simulink model "ChiefMaster_TTC580"  (R2022b)
settings: Solver=FixedStepAuto  StartTime=0.0  StopTime=10  FixedStep=0.01  RelTol=1e-3
values from neighbouring files (symbols this model uses):
  BattBox1_No = single(1)    [Parameters.m]
  BattBox2_No = single(2)    [Parameters.m]
  BattBox3_No = single(3)    [Parameters.m]
  CurrentLB = single(-3)    [Parameters.m]
  CurrentReductionConstant_Lvl0 = single(0.03)    [Parameters.m]
  CurrentReductionConstant_Lvl1 = single(0.05)    [Parameters.m]
  CurrentReductionConstant_Lvl2 = single(0.07)    [Parameters.m]
  CurrentReductionConstant_Lvl3 = single(0.1)    [Parameters.m]
  CurrentUB = single(3)    [Parameters.m]
  DCHV_Minus_In_Delay_ms = single(500)    [Parameters.m]
  FL_sHVC_CellBalanceVoltage_mV = single(3500)    [Parameters.m]
  FL_sInrushCurrent_dividebyzero = single(0.00001)    [Parameters.m]
  FL_u8HMI_BuzzerTimer = uint8(3)    [Parameters.m]
  IP_boActValue = true    [Parameters.m]
  IP_boDeactValue = false    [Parameters.m]
  IP_boInitValue = false    [Parameters.m]
  IP_s_LB = 18000    [Parameters.m]
  IP_s_UB = 22000    [Parameters.m]
  IP_sBatt1_ChargeCurrentMax_Factor = single(0.1)    [Parameters.m]
  IP_sBatt1_ChargeCurrentMax_LB = single(0)    [Parameters.m]
  IP_sBatt1_ChargeCurrentMax_Offset = single(0)    [Parameters.m]
  IP_sBatt1_ChargeCurrentMax_UB = single(6553.5)    [Parameters.m]
  IP_sBatt1_Current_Factor = single(0.1)    [Parameters.m]
  IP_sBatt1_Current_LB = single(-3276.8)    [Parameters.m]
  IP_sBatt1_Current_Offset = single(0)    [Parameters.m]
  IP_sBatt1_Current_UB = single(3276.8)    [Parameters.m]
  IP_sBatt1_DisChargeCurrentMax_Factor = single(0.1)    [Parameters.m]
  IP_sBatt1_DisChargeCurrentMax_LB = single(0)    [Parameters.m]
  IP_sBatt1_DisChargeCurrentMax_Offset = single(0)    [Parameters.m]
  IP_sBatt1_DisChargeCurrentMax_UB = single(6553.5)    [Parameters.m]
  IP_sBatt1_InsulationResistance_Factor = single(5)    [Parameters.m]
  IP_sBatt1_InsulationResistance_LB = single(0)    [Parameters.m]
  IP_sBatt1_InsulationResistance_Offset = single(0)    [Parameters.m]
  IP_sBatt1_InsulationResistance_UB = single(0)    [Parameters.m]
  IP_sBatt1_LiBa_IntResist_mOhm = single(25)    [Parameters.m]
  IP_sBatt1_SOC_Factor = single(1)    [Parameters.m]
  IP_sBatt1_SOC_LB = single(0)    [Parameters.m]
  IP_sBatt1_SOC_Offset = single(0)    [Parameters.m]
  IP_sBatt1_SOC_UB = single(100)    [Parameters.m]
  IP_sBatt1_SOH_Factor = single(1)    [Parameters.m]
  IP_sBatt1_SOH_LB = single(0)    [Parameters.m]
  IP_sBatt1_SOH_Offset = single(0)    [Parameters.m]
  IP_sBatt1_SOH_UB = single(100)    [Parameters.m]
  IP_sBatt1_Ubatt_Factor = single(0.1)    [Parameters.m]
  IP_sBatt1_Ubatt_LB = single(0)    [Parameters.m]
  IP_sBatt1_Ubatt_Offset = single(0)    [Parameters.m]
  IP_sBatt1_Ubatt_UB = single(6553.5)    [Parameters.m]
  IP_sBatt1_UserRi_Factor = single(1)    [Parameters.m]
  IP_sBatt1_UserRi_LB = single(0)    [Parameters.m]
  IP_sBatt1_UserRi_Offset = single(0)    [Parameters.m]
  IP_sBatt1_UserRi_UB = single(255)    [Parameters.m]
  IP_sBatt1_VoltageAtSensor_Factor = single(0.02)    [Parameters.m]
  IP_sBatt1_VoltageAtSensor_LB = single(0)    [Parameters.m]
  IP_sBatt1_VoltageAtSensor_Offset = single(0)    [Parameters.m]
  IP_sBatt1_VoltageAtSensor_UB = single(1310.7)    [Parameters.m]
  IP_sBatt2_LiBa_IntResist_mOhm = single(25)    [Parameters.m]
  IP_sBatt3_LiBa_IntResist_mOhm = single(25)    [Parameters.m]
  IP_sEM_LB = 2000    [Parameters.m]
  IP_sEM_UB = 8000    [Parameters.m]
  IP_sFB_LB = 5000    [Parameters.m]
  IP_sFB_UB = 10000    [Parameters.m]
  IP_sHVIL_LB = 12000    [Parameters.m]
  IP_sHVIL_UB = 15000    [Parameters.m]
  IP_sLoad_Voltage_Factor = single(1)    [Parameters.m]
  IP_sLoad_Voltage_LB = single(0)    [Parameters.m]
  IP_sLoad_Voltage_Offset = single(0)    [Parameters.m]
  IP_sLoad_Voltage_UB = single(65535)    [Parameters.m]
  IP_u8HVIL_Delay_ms = uint8(100)    [Parameters.m]
  IP_u8HW_IN_delay_ms = uint8(100)    [Parameters.m]
  IT_sInsulationSafeValue_kOhm = single(650)    [Parameters.m]
  IT_u8IMD_DelayTime_s = uint8(20)    [Parameters.m]
  MainHV_Minus_In_Delay = single(5)    [Parameters.m]
  MainHV_StatusDelay = single(5)    [Parameters.m]
  NotAvailable_uint16 = single(65535)    [Parameters.m]
  NotAvailable_uint8 = uint8(255)    [Parameters.m]
  OP_boHVIL_Supply = boolean(1)    [Parameters.m]
  SafeCurrentToCloseHV_A = single(5)    [Parameters.m]
  SafeVoltageToCloseHV_V = single(0.5)    [Parameters.m]
  UnexpectedBattChargingFcn_Available = boolean(1)    [Parameters.m]
  Voltage_NA_UB = uint16(65535)    [Parameters.m]
  VoltageSensorAvailableBB1 = boolean(0)    [Parameters.m]
  VoltageSensorAvailableBB2 = boolean(0)    [Parameters.m]
  VoltageSensorAvailableBB3 = boolean(0)    [Parameters.m]
libraries: simulink x184, Library_DataProcessing_v1_1 x167, Library_DataProcessing_v1 x142, libCM x28
(part 12 of 19)

== system ChiefMaster_TTC580/ChiefMaster/Input Translation/Battery Signals/Subsystem10/Subsystem3 ==
  <IP_boBatt1_IMD_Active : Inport
  "IMD_Req_Databus  " : Inport  Port=2
  Bus Selector : BusSelector  OutputSignals=FL_IMD_Control_Databus.FL_boREQ_IMD_ON_BB1
  Constant : Constant  Value=0  OutDataTypeStr=boolean
  Delay : Delay  DelayLength=3
  Multiport Switch : MultiPortSwitch  DataPortForDefault=Additional data port  DiagnosticForDefault=Warning  SaturateOnIntegerOverflow=off  InputSameDT=off
  IP_boBMS_IMD_Active_BB1 : Outport  OutDataTypeStr=boolean
  wires:
  Multiport Switch/1 -> IP_boBMS_IMD_Active_BB1/1  "IP_boBMS_IMD_Active_BB1"
  <IP_boBatt1_IMD_Active/1 -> Multiport Switch/2
  [Select_Battery1] -> Multiport Switch/1
  Delay/1 -> Multiport Switch/3
  Constant/1 -> Multiport Switch/4, Multiport Switch/5
  "IMD_Req_Databus  "/1 -> Bus Selector/1
  Bus Selector/1 -> Delay/1  "<FL_boREQ_IMD_ON_BB1>"

== system ChiefMaster_TTC580/ChiefMaster/Input Translation/Battery Signals/Subsystem11/Subsystem1 ==
  <IP_sBatt2_UserRi_mOhms_DataBus> : Inport
  Bus Selector7 : BusSelector  OutputSignals=sData
  Constant : Constant  Value=0  OutDataTypeStr=single
  Constant1 : Constant  Value=IP_sBatt2_LiBa_IntResist_mOhm  OutDataTypeStr=single
  Multiport Switch : MultiPortSwitch  DataPortForDefault=Additional data port  DiagnosticForDefault=Warning  SaturateOnIntegerOverflow=off  InputSameDT=off
  IP_sBMS_InternalResistance_BB2 : Outport
  wires:
  Constant1/1 -> Multiport Switch/3
  <IP_sBatt2_UserRi_mOhms_DataBus>/1 -> Bus Selector7/1
  Multiport Switch/1 -> IP_sBMS_InternalResistance_BB2/1  "IP_sBMS_InternalResistance_BB2"
  [Select_Battery2] -> Multiport Switch/1
  Constant/1 -> Multiport Switch/5, Multiport Switch/4
  Bus Selector7/1 -> Multiport Switch/2  "<sData>"

== system ChiefMaster_TTC580/ChiefMaster/Input Translation/Battery Signals/Subsystem11/Subsystem2 ==
  <IP_sBatt3_UserRi_mOhms_DataBus> : Inport
  Bus Selector7 : BusSelector  OutputSignals=sData
  Constant : Constant  Value=0  OutDataTypeStr=single
  Constant1 : Constant  Value=IP_sBatt3_LiBa_IntResist_mOhm  OutDataTypeStr=single
  Multiport Switch : MultiPortSwitch  DataPortForDefault=Additional data port  DiagnosticForDefault=Warning  SaturateOnIntegerOverflow=off  InputSameDT=off
  IP_sBMS_InternalResistance_BB3 : Outport
  wires:
  Bus Selector7/1 -> Multiport Switch/2  "<sData>"
  Constant/1 -> Multiport Switch/4, Multiport Switch/5
  [Select_Battery3] -> Multiport Switch/1
  Multiport Switch/1 -> IP_sBMS_InternalResistance_BB3/1  "IP_sBMS_InternalResistance_BB3"
  <IP_sBatt3_UserRi_mOhms_DataBus>/1 -> Bus Selector7/1
  Constant1/1 -> Multiport Switch/3

== system ChiefMaster_TTC580/ChiefMaster/Input Translation/Battery Signals/Subsystem11/Subsystem3 ==
  <IP_sBatt1_UserRi_mOhms_DataBus> : Inport
  Bus Selector7 : BusSelector  OutputSignals=sData
  Constant : Constant  Value=0  OutDataTypeStr=single
  Constant1 : Constant  Value=IP_sBatt1_LiBa_IntResist_mOhm  OutDataTypeStr=single
  Multiport Switch : MultiPortSwitch  DataPortForDefault=Additional data port  DiagnosticForDefault=Warning  SaturateOnIntegerOverflow=off  InputSameDT=off
  IP_sBMS_InternalResistance_BB1 : Outport
  wires:
  Bus Selector7/1 -> Multiport Switch/2  "<sData>"
  Constant/1 -> Multiport Switch/4, Multiport Switch/5
  [Select_Battery1] -> Multiport Switch/1
  Multiport Switch/1 -> IP_sBMS_InternalResistance_BB1/1  "IP_sBMS_InternalResistance_BB1"
  <IP_sBatt1_UserRi_mOhms_DataBus>/1 -> Bus Selector7/1
  Constant1/1 -> Multiport Switch/3

== system ChiefMaster_TTC580/ChiefMaster/Input Translation/Battery Signals/Subsystem12/Subsystem1 ==
  <IP_sBatt2_InsulationResistance_kOhms_DataBus> : Inport
  <IP_LB_BMS_Pack_Leak_Pos_Raw_mV_DataBus> : Inport  Port=2
  <IP_LB_BMS_Pack_Leak_Neg_Raw_mV_DataBus> : Inport  Port=3
  <IP_LB_BMS_Pack_V_Cells_DataBus> : Inport  Port=4
  Bus Selector : BusSelector  OutputSignals=sData
  Constant : Constant  Value=0  OutDataTypeStr=single
  Multiport Switch : MultiPortSwitch  DataPortForDefault=Additional data port  DiagnosticForDefault=Warning  SaturateOnIntegerOverflow=off  InputSameDT=off
  Subsystem1 : Subsystem
  IP_boBMS_InsulationResistance_kOhm_BB1 : Outport  OutDataTypeStr=single
  IP_boBMS_InsulationResistance_Minus_kOhm_BB1 : Outport  Port=2  OutDataTypeStr=single
  IP_LiBa_Insulation_OK_BB1 : Outport  Port=3
  wires:
  Bus Selector/1 -> Multiport Switch/2  "<sData>"
  <IP_sBatt2_InsulationResistance_kOhms_DataBus>/1 -> Bus Selector/1
  Multiport Switch/1 -> IP_boBMS_InsulationResistance_kOhm_BB1/1  "IP_boBMS_InsulationResistance_kOhm_B2"
  [Select_Battery2] -> Multiport Switch/1
  <IP_LB_BMS_Pack_V_Cells_DataBus>/1 -> Subsystem1/3(<IP_LB_BMS_Pack_V_Cells_DataBus>)
  Subsystem1/1(IP_sLiBa_InsulationRes_Plus_kOhm) -> Multiport Switch/3
  Constant/1 -> Multiport Switch/4, Multiport Switch/5
  <IP_LB_BMS_Pack_Leak_Pos_Raw_mV_DataBus>/1 -> Subsystem1/1(<IP_LB_BMS_Pack_Leak_Pos_Raw_mV_DataBus>)
  <IP_LB_BMS_Pack_Leak_Neg_Raw_mV_DataBus>/1 -> Subsystem1/2(<IP_LB_BMS_Pack_Leak_Neg_Raw_mV_DataBus>)
  Subsystem1/2(IP_sLiBa_InsulationRes_Minus_kOhm) -> IP_boBMS_InsulationResistance_Minus_kOhm_BB1/1
  Subsystem1/3(IP_LiBa_Insulation_Ok_Batt) -> IP_LiBa_Insulation_OK_BB1/1

== system ChiefMaster_TTC580/ChiefMaster/Input Translation/Battery Signals/Subsystem12/Subsystem2 ==
  <IP_sBatt3_InsulationResistance_kOhms_DataBus> : Inport
  <IP_LB_BMS_Pack_Leak_Pos_Raw_mV_DataBus> : Inport  Port=2
  <IP_LB_BMS_Pack_Leak_Neg_Raw_mV_DataBus> : Inport  Port=3
  <IP_LB_BMS_Pack_V_Cells_DataBus> : Inport  Port=4
  Bus Selector : BusSelector  OutputSignals=sData
  Constant : Constant  Value=0  OutDataTypeStr=single
  Multiport Switch : MultiPortSwitch  DataPortForDefault=Additional data port  DiagnosticForDefault=Warning  SaturateOnIntegerOverflow=off  InputSameDT=off
  Subsystem1 : Subsystem
  IP_boBMS_InsulationResistance_kOhm_B3 : Outport  OutDataTypeStr=single
  IP_sLiBa_InsulationRes_Minus_BB3_kOhm : Outport  Port=2  OutDataTypeStr=single
  IP_LiBa_Insulation_Ok_Batt3 : Outport  Port=3
  wires:
  <IP_LB_BMS_Pack_Leak_Pos_Raw_mV_DataBus>/1 -> Subsystem1/1(<IP_LB_BMS_Pack_Leak_Pos_Raw_mV_DataBus>)
  Constant/1 -> Multiport Switch/5, Multiport Switch/4
  Subsystem1/1(IP_sLiBa_InsulationRes_Plus_kOhm) -> Multiport Switch/3
  <IP_LB_BMS_Pack_V_Cells_DataBus>/1 -> Subsystem1/3(<IP_LB_BMS_Pack_V_Cells_DataBus>)
  [Select_Battery3] -> Multiport Switch/1
  Multiport Switch/1 -> IP_boBMS_InsulationResistance_kOhm_B3/1  "IP_boBMS_InsulationResistance_kOhm_B3"
  <IP_sBatt3_InsulationResistance_kOhms_DataBus>/1 -> Bus Selector/1
  Bus Selector/1 -> Multiport Switch/2  "<sData>"
  <IP_LB_BMS_Pack_Leak_Neg_Raw_mV_DataBus>/1 -> Subsystem1/2(<IP_LB_BMS_Pack_Leak_Neg_Raw_mV_DataBus>)
  Subsystem1/3(IP_LiBa_Insulation_Ok_Batt) -> IP_LiBa_Insulation_Ok_Batt3/1
  Subsystem1/2(IP_sLiBa_InsulationRes_Minus_kOhm) -> IP_sLiBa_InsulationRes_Minus_BB3_kOhm/1

== system ChiefMaster_TTC580/ChiefMaster/Input Translation/Battery Signals/Subsystem12/Subsystem3 ==
  <IP_sBatt1_InsulationResistance_kOhms_DataBus> : Inport
  <IP_LB_BMS_Pack_Leak_Pos_Raw_mV_DataBus> : Inport  Port=2
  <IP_LB_BMS_Pack_Leak_Neg_Raw_mV_DataBus> : Inport  Port=3
  <IP_LB_BMS_Pack_V_Cells_DataBus> : Inport  Port=4
  Bus Selector : BusSelector  OutputSignals=sData
  Constant : Constant  Value=0  OutDataTypeStr=single
  Multiport Switch : MultiPortSwitch  DataPortForDefault=Additional data port  DiagnosticForDefault=Warning  SaturateOnIntegerOverflow=off  InputSameDT=off
  Subsystem1 : Subsystem
  IP_boBMS_InsulationResistance_kOhm_BB1 : Outport  OutDataTypeStr=single
  IP_boBMS_InsulationResistance_Minus_kOhm_BB1 : Outport  Port=2  OutDataTypeStr=single
  IP_LiBa_Insulation_OK_BB1 : Outport  Port=3
  wires:
  <IP_LB_BMS_Pack_Leak_Pos_Raw_mV_DataBus>/1 -> Subsystem1/1(<IP_LB_BMS_Pack_Leak_Pos_Raw_mV_DataBus>)
  Constant/1 -> Multiport Switch/5, Multiport Switch/4
  <IP_LB_BMS_Pack_V_Cells_DataBus>/1 -> Subsystem1/3(<IP_LB_BMS_Pack_V_Cells_DataBus>)
  [Select_Battery1] -> Multiport Switch/1
  Multiport Switch/1 -> IP_boBMS_InsulationResistance_kOhm_BB1/1  "IP_boBMS_InsulationResistance_kOhm_BB1"
  <IP_sBatt1_InsulationResistance_kOhms_DataBus>/1 -> Bus Selector/1
  Bus Selector/1 -> Multiport Switch/2  "<sData>"
  <IP_LB_BMS_Pack_Leak_Neg_Raw_mV_DataBus>/1 -> Subsystem1/2(<IP_LB_BMS_Pack_Leak_Neg_Raw_mV_DataBus>)
  Subsystem1/1(IP_sLiBa_InsulationRes_Plus_kOhm) -> Multiport Switch/3
  Subsystem1/2(IP_sLiBa_InsulationRes_Minus_kOhm) -> IP_boBMS_InsulationResistance_Minus_kOhm_BB1/1  "IP_sLiBa_InsulationRes_Minus_BB1_kOhm"
  Subsystem1/3(IP_LiBa_Insulation_Ok_Batt) -> IP_LiBa_Insulation_OK_BB1/1

== system ChiefMaster_TTC580/ChiefMaster/Input Translation/Battery Signals/Subsystem14/Subsystem1 ==
  <IP_sActia_Batt2_MinCellVolt_DataBus> : Inport
  <IP_LB_BMS_ACT_Cel_mV_Min_DataBus> : Inport  Port=2
  Bus Selector1 : BusSelector  OutputSignals=sData
  Bus Selector7 : BusSelector  OutputSignals=sData
  Constant : Constant  Value=0  OutDataTypeStr=single
  Multiport Switch : MultiPortSwitch  DataPortForDefault=Additional data port  DiagnosticForDefault=Warning  SaturateOnIntegerOverflow=off  InputSameDT=off
  IP_sBMS_MinCellVoltage_BB2 : Outport
  wires:
  Multiport Switch/1 -> IP_sBMS_MinCellVoltage_BB2/1  "IP_sBMS_MinCellVoltage_BB2"
  [Select_Battery2] -> Multiport Switch/1
  Constant/1 -> Multiport Switch/5, Multiport Switch/4
  <IP_sActia_Batt2_MinCellVolt_DataBus>/1 -> Bus Selector1/1
  <IP_LB_BMS_ACT_Cel_mV_Min_DataBus>/1 -> Bus Selector7/1
  Bus Selector7/1 -> Multiport Switch/3  "<sData>"
  Bus Selector1/1 -> Multiport Switch/2  "<sData>"

== system ChiefMaster_TTC580/ChiefMaster/Input Translation/Battery Signals/Subsystem14/Subsystem2 ==
  <IP_sActia_Batt3_MinCellVolt_DataBus> : Inport
  <IP_LB_BMS_ACT_Cel_mV_Min_DataBus> : Inport  Port=2
  Bus Selector1 : BusSelector  OutputSignals=sData
  Bus Selector7 : BusSelector  OutputSignals=sData
  Constant : Constant  Value=0  OutDataTypeStr=single
  Multiport Switch : MultiPortSwitch  DataPortForDefault=Additional data port  DiagnosticForDefault=Warning  SaturateOnIntegerOverflow=off  InputSameDT=off
  IP_sBMS_MinCellVoltage_BB3 : Outport
  wires:
  Bus Selector1/1 -> Multiport Switch/2  "<sData>"
  Bus Selector7/1 -> Multiport Switch/3  "<sData>"
  <IP_LB_BMS_ACT_Cel_mV_Min_DataBus>/1 -> Bus Selector7/1
  <IP_sActia_Batt3_MinCellVolt_DataBus>/1 -> Bus Selector1/1
  Constant/1 -> Multiport Switch/4, Multiport Switch/5
  [Select_Battery3] -> Multiport Switch/1
  Multiport Switch/1 -> IP_sBMS_MinCellVoltage_BB3/1  "IP_sBMS_MinCellVoltage_BB3"

== system ChiefMaster_TTC580/ChiefMaster/Input Translation/Battery Signals/Subsystem14/Subsystem3 ==
  <IP_sActia_Batt1_MinCellVolt_mV_DataBus> : Inport
  <IP_LB_BMS_ACT_Cel_mV_Min_DataBus> : Inport  Port=2
  Bus Selector1 : BusSelector  OutputSignals=sData
  Bus Selector7 : BusSelector  OutputSignals=sData
  Constant : Constant  Value=0  OutDataTypeStr=single
  Multiport Switch : MultiPortSwitch  DataPortForDefault=Additional data port  DiagnosticForDefault=Warning  SaturateOnIntegerOverflow=off  InputSameDT=off
  IP_sBMS_MinCellVoltage_BB1 : Outport
  wires:
  Bus Selector1/1 -> Multiport Switch/2  "<sData>"
  Bus Selector7/1 -> Multiport Switch/3  "<sData>"
  <IP_LB_BMS_ACT_Cel_mV_Min_DataBus>/1 -> Bus Selector7/1
  <IP_sActia_Batt1_MinCellVolt_mV_DataBus>/1 -> Bus Selector1/1
  Constant/1 -> Multiport Switch/4, Multiport Switch/5
  [Select_Battery1] -> Multiport Switch/1
  Multiport Switch/1 -> IP_sBMS_MinCellVoltage_BB1/1  "IP_sBMS_MinCellVoltage_BB1"

== system ChiefMaster_TTC580/ChiefMaster/Input Translation/Battery Signals/Subsystem14/Subsystem4 ==
  <IP_sActia_Batt2_MaxCellVolt_DataBus> : Inport
  <IP_LB_BMS_ACT_Cel_mV_Min_DataBus> : Inport  Port=2
  Bus Selector1 : BusSelector  OutputSignals=sData
  Bus Selector7 : BusSelector  OutputSignals=sData
  Constant : Constant  Value=0  OutDataTypeStr=single
  Multiport Switch : MultiPortSwitch  DataPortForDefault=Additional data port  DiagnosticForDefault=Warning  SaturateOnIntegerOverflow=off  InputSameDT=off
  IP_sBMS_MaxCellVoltage_BB2 : Outport
  wires:
  Bus Selector1/1 -> Multiport Switch/2  "<sData>"
  Bus Selector7/1 -> Multiport Switch/3  "<sData>"
  <IP_LB_BMS_ACT_Cel_mV_Min_DataBus>/1 -> Bus Selector7/1
  <IP_sActia_Batt2_MaxCellVolt_DataBus>/1 -> Bus Selector1/1
  Constant/1 -> Multiport Switch/4, Multiport Switch/5
  [Select_Battery2] -> Multiport Switch/1
  Multiport Switch/1 -> IP_sBMS_MaxCellVoltage_BB2/1  "IP_sBMS_MaxCellVoltage_BB2"

== system ChiefMaster_TTC580/ChiefMaster/Input Translation/Battery Signals/Subsystem14/Subsystem5 ==
  <IP_sActia_Batt3_MaxCellVolt_DataBus> : Inport
  <IP_LB_BMS_ACT_Cel_mV_Min_DataBus> : Inport  Port=2
  Bus Selector1 : BusSelector  OutputSignals=sData
  Bus Selector7 : BusSelector  OutputSignals=sData
  Constant : Constant  Value=0  OutDataTypeStr=single
  Multiport Switch : MultiPortSwitch  DataPortForDefault=Additional data port  DiagnosticForDefault=Warning  SaturateOnIntegerOverflow=off  InputSameDT=off
  IP_sBMS_MaxCellVoltage_BB3 : Outport
  wires:
  Multiport Switch/1 -> IP_sBMS_MaxCellVoltage_BB3/1  "IP_sBMS_MaxCellVoltage_BB3"
  [Select_Battery3] -> Multiport Switch/1
  Constant/1 -> Multiport Switch/5, Multiport Switch/4
  <IP_sActia_Batt3_MaxCellVolt_DataBus>/1 -> Bus Selector1/1
  <IP_LB_BMS_ACT_Cel_mV_Min_DataBus>/1 -> Bus Selector7/1
  Bus Selector1/1 -> Multiport Switch/2  "<sData>"
  Bus Selector7/1 -> Multiport Switch/3  "<sData>"

== system ChiefMaster_TTC580/ChiefMaster/Input Translation/Battery Signals/Subsystem14/Subsystem6 ==
  <IP_sActia_Batt1_MaxCellVolt_DataBus> : Inport
  <IP_LB_BMS_ACT_Cel_mV_Min_DataBus> : Inport  Port=2
  Bus Selector1 : BusSelector  OutputSignals=sData
  Bus Selector7 : BusSelector  OutputSignals=sData
  Constant : Constant  Value=0  OutDataTypeStr=single
  Multiport Switch : MultiPortSwitch  DataPortForDefault=Additional data port  DiagnosticForDefault=Warning  SaturateOnIntegerOverflow=off  InputSameDT=off
  IP_sBMS_MaxCellVoltage_BB1 : Outport
  wires:
  Multiport Switch/1 -> IP_sBMS_MaxCellVoltage_BB1/1  "IP_sBMS_MaxCellVoltage_BB1"
  [Select_Battery1] -> Multiport Switch/1
  Constant/1 -> Multiport Switch/5, Multiport Switch/4
  <IP_sActia_Batt1_MaxCellVolt_DataBus>/1 -> Bus Selector1/1
  <IP_LB_BMS_ACT_Cel_mV_Min_DataBus>/1 -> Bus Selector7/1
  Bus Selector1/1 -> Multiport Switch/2  "<sData>"
  Bus Selector7/1 -> Multiport Switch/3  "<sData>"

== system ChiefMaster_TTC580/ChiefMaster/Input Translation/Battery Signals/Subsystem15/Subsystem1 ==
  <IP_sActia_Batt1_MaxTemp_degC_DataBus> : Inport
  <IP_LB_BMS_ACT_Cel_T_Max_Value_DataBus> : Inport  Port=2
  Bus Selector1 : BusSelector  OutputSignals=sData
  Bus Selector7 : BusSelector  OutputSignals=sData
  Constant : Constant  Value=0  OutDataTypeStr=single
  Multiport Switch : MultiPortSwitch  DataPortForDefault=Additional data port  DiagnosticForDefault=Warning  SaturateOnIntegerOverflow=off  InputSameDT=off
  IP_sBMS_MaxTemp_degC_BB1 : Outport
  wires:
  <IP_LB_BMS_ACT_Cel_T_Max_Value_DataBus>/1 -> Bus Selector1/1
  <IP_sActia_Batt1_MaxTemp_degC_DataBus>/1 -> Bus Selector7/1
  Bus Selector1/1 -> Multiport Switch/3  "<sData>"
  Bus Selector7/1 -> Multiport Switch/2  "<sData>"
  Constant/1 -> Multiport Switch/4, Multiport Switch/5
  [Select_Battery1] -> Multiport Switch/1
  Multiport Switch/1 -> IP_sBMS_MaxTemp_degC_BB1/1  "IP_sBMS_MaxTemp_degC_BB1"

== system ChiefMaster_TTC580/ChiefMaster/Input Translation/Battery Signals/Subsystem15/Subsystem2 ==
  <IP_sActia_Batt2_MinTemp_degC_DataBus> : Inport
  <IP_LB_BMS_ACT_Cel_T_Min_Value_DataBus> : Inport  Port=2
  Bus Selector1 : BusSelector  OutputSignals=sData
  Bus Selector7 : BusSelector  OutputSignals=sData
  Constant : Constant  Value=0  OutDataTypeStr=single
  Multiport Switch : MultiPortSwitch  DataPortForDefault=Additional data port  DiagnosticForDefault=Warning  SaturateOnIntegerOverflow=off  InputSameDT=off
  IP_sBMS_MinTemp_degC_BB2 : Outport
  wires:
  <IP_LB_BMS_ACT_Cel_T_Min_Value_DataBus>/1 -> Bus Selector1/1
  <IP_sActia_Batt2_MinTemp_degC_DataBus>/1 -> Bus Selector7/1
  Bus Selector7/1 -> Multiport Switch/2  "<sData>"
  Bus Selector1/1 -> Multiport Switch/3  "<sData>"
  [Select_Battery2] -> Multiport Switch/1
  Multiport Switch/1 -> IP_sBMS_MinTemp_degC_BB2/1  "IP_sBMS_MinTemp_degC_BB2"
  Constant/1 -> Multiport Switch/4, Multiport Switch/5

== system ChiefMaster_TTC580/ChiefMaster/Input Translation/Battery Signals/Subsystem15/Subsystem3 ==
  <IP_sActia_Batt1_MinTemp_degC_DataBus> : Inport
  <IP_LB_BMS_ACT_Cel_T_Min_Value_DataBus> : Inport  Port=2
  Bus Selector1 : BusSelector  OutputSignals=sData
  Bus Selector7 : BusSelector  OutputSignals=sData
  Constant : Constant  Value=0  OutDataTypeStr=single
  Multiport Switch : MultiPortSwitch  DataPortForDefault=Additional data port  DiagnosticForDefault=Warning  SaturateOnIntegerOverflow=off  InputSameDT=off
  IP_sBMS_MinTemp_degC_BB1 : Outport
  wires:
  Multiport Switch/1 -> IP_sBMS_MinTemp_degC_BB1/1  "IP_sBMS_MinTemp_degC_BB1"
  [Select_Battery1] -> Multiport Switch/1
  Constant/1 -> Multiport Switch/5, Multiport Switch/4
  Bus Selector7/1 -> Multiport Switch/2  "<sData>"
  Bus Selector1/1 -> Multiport Switch/3  "<sData>"
  <IP_sActia_Batt1_MinTemp_degC_DataBus>/1 -> Bus Selector7/1
  <IP_LB_BMS_ACT_Cel_T_Min_Value_DataBus>/1 -> Bus Selector1/1

== system ChiefMaster_TTC580/ChiefMaster/Input Translation/Battery Signals/Subsystem15/Subsystem4 ==
  <IP_sActia_Batt2_MaxTemp_degC_DataBus> : Inport
  <IP_LB_BMS_ACT_Cel_T_Max_Value_DataBus> : Inport  Port=2
  Bus Selector1 : BusSelector  OutputSignals=sData
  Bus Selector7 : BusSelector  OutputSignals=sData
  Constant : Constant  Value=0  OutDataTypeStr=single
  Multiport Switch : MultiPortSwitch  DataPortForDefault=Additional data port  DiagnosticForDefault=Warning  SaturateOnIntegerOverflow=off  InputSameDT=off
  IP_sBMS_MaxTemp_degC_BB2 : Outport
  wires:
  Multiport Switch/1 -> IP_sBMS_MaxTemp_degC_BB2/1  "IP_sBMS_MaxTemp_degC_BB2"
  [Select_Battery2] -> Multiport Switch/1
  Constant/1 -> Multiport Switch/5, Multiport Switch/4
  Bus Selector7/1 -> Multiport Switch/2  "<sData>"
  Bus Selector1/1 -> Multiport Switch/3  "<sData>"
  <IP_sActia_Batt2_MaxTemp_degC_DataBus>/1 -> Bus Selector7/1
  <IP_LB_BMS_ACT_Cel_T_Max_Value_DataBus>/1 -> Bus Selector1/1

== system ChiefMaster_TTC580/ChiefMaster/Input Translation/Battery Signals/Subsystem15/Subsystem5 ==
  <IP_sActia_Batt3_MinTemp_degC_DataBus> : Inport
  <IP_LB_BMS_ACT_Cel_T_Min_Value_DataBus> : Inport  Port=2
  Bus Selector1 : BusSelector  OutputSignals=sData
  Bus Selector7 : BusSelector  OutputSignals=sData
  Constant : Constant  Value=0  OutDataTypeStr=single
  Multiport Switch : MultiPortSwitch  DataPortForDefault=Additional data port  DiagnosticForDefault=Warning  SaturateOnIntegerOverflow=off  InputSameDT=off
  IP_sBMS_MinTemp_degC_BB3 : Outport
  wires:
  Multiport Switch/1 -> IP_sBMS_MinTemp_degC_BB3/1  "IP_sBMS_MinTemp_degC_BB3"
  [Select_Battery3] -> Multiport Switch/1
  Constant/1 -> Multiport Switch/5, Multiport Switch/4
  Bus Selector7/1 -> Multiport Switch/2  "<sData>"
  Bus Selector1/1 -> Multiport Switch/3  "<sData>"
  <IP_sActia_Batt3_MinTemp_degC_DataBus>/1 -> Bus Selector7/1
  <IP_LB_BMS_ACT_Cel_T_Min_Value_DataBus>/1 -> Bus Selector1/1

== system ChiefMaster_TTC580/ChiefMaster/Input Translation/Battery Signals/Subsystem15/Subsystem6 ==
  <IP_sActia_Batt3_MaxTemp_degC_DataBus> : Inport
  <IP_LB_BMS_ACT_Cel_T_Max_Value_DataBus> : Inport  Port=2
  Bus Selector1 : BusSelector  OutputSignals=sData
  Bus Selector7 : BusSelector  OutputSignals=sData
  Constant : Constant  Value=0  OutDataTypeStr=single
  Multiport Switch : MultiPortSwitch  DataPortForDefault=Additional data port  DiagnosticForDefault=Warning  SaturateOnIntegerOverflow=off  InputSameDT=off
  IP_sBMS_MaxTemp_degC_BB3 : Outport
  wires:
  <IP_LB_BMS_ACT_Cel_T_Max_Value_DataBus>/1 -> Bus Selector1/1
  <IP_sActia_Batt3_MaxTemp_degC_DataBus>/1 -> Bus Selector7/1
  Bus Selector1/1 -> Multiport Switch/3  "<sData>"
  Bus Selector7/1 -> Multiport Switch/2  "<sData>"
  Constant/1 -> Multiport Switch/4, Multiport Switch/5
  [Select_Battery3] -> Multiport Switch/1
  Multiport Switch/1 -> IP_sBMS_MaxTemp_degC_BB3/1  "IP_sBMS_MaxTemp_degC_BB3"

== system ChiefMaster_TTC580/ChiefMaster/Input Translation/Battery Signals/Subsystem2/Subsystem ==
  IP_boBatt1_HV_REL_ON : Inport
  IP_LB_BMS_IO_state_Input_DataBus : Inport  Port=2
  Bus Selector : BusSelector  OutputSignals=sData
  Compare To Constant : simulink/Logic and Bit Operations/Compare To Constant  relop===  const=192  OutDataTypeStr=boolean
  Compare To Constant2 : simulink/Logic and Bit Operations/Compare To Constant  relop===  const=224  OutDataTypeStr=boolean
  Constant : Constant  Value=0  OutDataTypeStr=boolean
  Multiport Switch : MultiPortSwitch  DataPortForDefault=Additional data port  DiagnosticForDefault=Warning  SaturateOnIntegerOverflow=off  InputSameDT=off
  OR : Logic  Operator=OR  AllPortsSameDT=off  OutDataTypeStr=boolean
  IP_boBMS_HV_REL_ON_BB1 : Outport
  wires:
  Multiport Switch/1 -> IP_boBMS_HV_REL_ON_BB1/1  "IP_boBMS_HV_REL_ON_BB1"
  [Select_Battery1] -> Multiport Switch/1
  Bus Selector/1 -> Compare To Constant/1, Compare To Constant2/1  "<sData>"
  Constant/1 -> Multiport Switch/4, Multiport Switch/5
  IP_boBatt1_HV_REL_ON/1 -> Multiport Switch/2
  IP_LB_BMS_IO_state_Input_DataBus/1 -> Bus Selector/1
  OR/1 -> Multiport Switch/3
  Compare To Constant2/1 -> OR/2
  Compare To Constant/1 -> OR/1

== system ChiefMaster_TTC580/ChiefMaster/Input Translation/Battery Signals/Subsystem2/Subsystem1 ==
  IP_boBatt2_HV_REL_ON : Inport
  IP_LB_BMS_IO_state_Input_DataBus : Inport  Port=2
  Bus Selector : BusSelector  OutputSignals=sData
  Compare To Constant : simulink/Logic and Bit Operations/Compare To Constant  relop===  const=192  OutDataTypeStr=boolean
  Compare To Constant2 : simulink/Logic and Bit Operations/Compare To Constant  relop===  const=224  OutDataTypeStr=boolean
  Constant : Constant  Value=0  OutDataTypeStr=boolean
  Multiport Switch : MultiPortSwitch  DataPortForDefault=Additional data port  DiagnosticForDefault=Warning  SaturateOnIntegerOverflow=off  InputSameDT=off
  OR : Logic  Operator=OR  AllPortsSameDT=off  OutDataTypeStr=boolean
  IP_boBMS_HV_REL_ON_BB2 : Outport
  wires:
  OR/1 -> Multiport Switch/3
  IP_LB_BMS_IO_state_Input_DataBus/1 -> Bus Selector/1
  IP_boBatt2_HV_REL_ON/1 -> Multiport Switch/2
  Constant/1 -> Multiport Switch/5, Multiport Switch/4
  Bus Selector/1 -> Compare To Constant/1, Compare To Constant2/1  "<sData>"
  [Select_Battery2] -> Multiport Switch/1
  Multiport Switch/1 -> IP_boBMS_HV_REL_ON_BB2/1  "IP_boBMS_HV_REL_ON_BB2"
  Compare To Constant/1 -> OR/1
  Compare To Constant2/1 -> OR/2

== system ChiefMaster_TTC580/ChiefMaster/Input Translation/Battery Signals/Subsystem2/Subsystem2 ==
  IP_boBatt3_HV_REL_ON : Inport
  IP_LB_BMS_IO_state_Input_DataBus : Inport  Port=2
  Bus Selector : BusSelector  OutputSignals=sData
  Compare To Constant : simulink/Logic and Bit Operations/Compare To Constant  relop===  const=192  OutDataTypeStr=boolean
  Compare To Constant2 : simulink/Logic and Bit Operations/Compare To Constant  relop===  const=224  OutDataTypeStr=boolean
  Constant : Constant  Value=0  OutDataTypeStr=boolean
  Multiport Switch : MultiPortSwitch  DataPortForDefault=Additional data port  DiagnosticForDefault=Warning  SaturateOnIntegerOverflow=off  InputSameDT=off
  OR : Logic  Operator=OR  AllPortsSameDT=off  OutDataTypeStr=boolean
  IP_boBMS_HV_REL_ON_BB3 : Outport
  wires:
  Multiport Switch/1 -> IP_boBMS_HV_REL_ON_BB3/1  "IP_boBMS_HV_REL_ON_BB3"
  [Select_Battery3] -> Multiport Switch/1
  Bus Selector/1 -> Compare To Constant2/1, Compare To Constant/1  "<sData>"
  Constant/1 -> Multiport Switch/4, Multiport Switch/5
  IP_boBatt3_HV_REL_ON/1 -> Multiport Switch/2
  IP_LB_BMS_IO_state_Input_DataBus/1 -> Bus Selector/1
  OR/1 -> Multiport Switch/3
  Compare To Constant/1 -> OR/1
  Compare To Constant2/1 -> OR/2

== system ChiefMaster_TTC580/ChiefMaster/Input Translation/Battery Signals/Subsystem3/Subsystem ==
  <IP_sBatt1_SOC_percent_DataBus> : Inport
  <IP_LB_BMS_Pack_Q_SOC_Internal_DataBus> : Inport  Port=2
  Bus Selector1 : BusSelector  OutputSignals=sData
  Bus Selector10 : BusSelector  OutputSignals=sData
  Constant : Constant  Value=0  OutDataTypeStr=single
  Multiport Switch : MultiPortSwitch  DataPortForDefault=Additional data port  DiagnosticForDefault=Warning  SaturateOnIntegerOverflow=off  InputSameDT=off
  IP_sBMS_SOC_BB1 : Outport
  wires:
  Multiport Switch/1 -> IP_sBMS_SOC_BB1/1  "IP_sBMS_SOC_BB1"
  Bus Selector10/1 -> Multiport Switch/2  "<sData>"
  Bus Selector1/1 -> Multiport Switch/3  "<sData>"
  <IP_LB_BMS_Pack_Q_SOC_Internal_DataBus>/1 -> Bus Selector1/1
  Constant/1 -> Multiport Switch/4, Multiport Switch/5
  [Select_Battery1] -> Multiport Switch/1
  <IP_sBatt1_SOC_percent_DataBus>/1 -> Bus Selector10/1

== system ChiefMaster_TTC580/ChiefMaster/Input Translation/Battery Signals/Subsystem3/Subsystem1 ==
  <IP_sBatt2_SOC_percent_DataBus> : Inport
  <IP_LB_BMS_Pack_Q_SOC_Internal_DataBus> : Inport  Port=2
  Bus Selector1 : BusSelector  OutputSignals=sData
  Bus Selector10 : BusSelector  OutputSignals=sData
  Constant : Constant  Value=0  OutDataTypeStr=single
  Multiport Switch : MultiPortSwitch  DataPortForDefault=Additional data port  DiagnosticForDefault=Warning  SaturateOnIntegerOverflow=off  InputSameDT=off
  IP_sBMS_SOC_BB2 : Outport
  wires:
  <IP_sBatt2_SOC_percent_DataBus>/1 -> Bus Selector10/1
  [Select_Battery2] -> Multiport Switch/1
  Constant/1 -> Multiport Switch/5, Multiport Switch/4
  <IP_LB_BMS_Pack_Q_SOC_Internal_DataBus>/1 -> Bus Selector1/1
  Bus Selector1/1 -> Multiport Switch/3  "<sData>"
  Bus Selector10/1 -> Multiport Switch/2  "<sData>"
  Multiport Switch/1 -> IP_sBMS_SOC_BB2/1  "IP_sBMS_SOC_BB2"

== system ChiefMaster_TTC580/ChiefMaster/Input Translation/Battery Signals/Subsystem3/Subsystem2 ==
  <IP_sBatt3_SOC_percent_DataBus> : Inport
  <IP_LB_BMS_Pack_Q_SOC_Internal_DataBus> : Inport  Port=2
  Bus Selector1 : BusSelector  OutputSignals=sData
  Bus Selector10 : BusSelector  OutputSignals=sData
  Constant : Constant  Value=0  OutDataTypeStr=single
  Multiport Switch : MultiPortSwitch  DataPortForDefault=Additional data port  DiagnosticForDefault=Warning  SaturateOnIntegerOverflow=off  InputSameDT=off
  IP_sBMS_SOC_BB3 : Outport
  wires:
  Multiport Switch/1 -> IP_sBMS_SOC_BB3/1  "IP_sBMS_SOC_BB3"
  Bus Selector10/1 -> Multiport Switch/2  "<sData>"
  Bus Selector1/1 -> Multiport Switch/3  "<sData>"
  <IP_LB_BMS_Pack_Q_SOC_Internal_DataBus>/1 -> Bus Selector1/1
  Constant/1 -> Multiport Switch/4, Multiport Switch/5
  [Select_Battery3] -> Multiport Switch/1
  <IP_sBatt3_SOC_percent_DataBus>/1 -> Bus Selector10/1

== system ChiefMaster_TTC580/ChiefMaster/Input Translation/Battery Signals/Subsystem4/Subsystem ==
  <IP_sBatt1_DisChargeCurrentMax_A_Databus> : Inport
  <IP_LB_BMS_DYN_Lim_Current_OUT_A_DataBus> : Inport  Port=2
  Bus Selector : BusSelector  OutputSignals=sData
  Bus Selector1 : BusSelector  OutputSignals=sData
  Constant : Constant  Value=0  OutDataTypeStr=single
  Multiport Switch : MultiPortSwitch  DataPortForDefault=Additional data port  DiagnosticForDefault=Warning  SaturateOnIntegerOverflow=off  InputSameDT=off
  IP_sBMS_DisChargeCurrentPrognosis_BB1 : Outport
  wires:
  Bus Selector/1 -> Multiport Switch/2  "<sData>"
  Multiport Switch/1 -> IP_sBMS_DisChargeCurrentPrognosis_BB1/1  "IP_sBMS_DisChargeCurrentPrognosis_BB1"
  Constant/1 -> Multiport Switch/4, Multiport Switch/5
  <IP_sBatt1_DisChargeCurrentMax_A_Databus>/1 -> Bus Selector/1
  [Select_Battery1] -> Multiport Switch/1
  Bus Selector1/1 -> Multiport Switch/3  "<sData>"
  <IP_LB_BMS_DYN_Lim_Current_OUT_A_DataBus>/1 -> Bus Selector1/1

== system ChiefMaster_TTC580/ChiefMaster/Input Translation/Battery Signals/Subsystem4/Subsystem1 ==
  <IP_sBatt2_DisChargeCurrentMax_A_Databus> : Inport
  <IP_LB_BMS_DYN_Lim_Current_OUT_A_DataBus> : Inport  Port=2
  Bus Selector : BusSelector  OutputSignals=sData
  Bus Selector1 : BusSelector  OutputSignals=sData
  Constant : Constant  Value=0  OutDataTypeStr=single
  Multiport Switch : MultiPortSwitch  DataPortForDefault=Additional data port  DiagnosticForDefault=Warning  SaturateOnIntegerOverflow=off  InputSameDT=off
  IP_sBMS_DisChargeCurrentPrognosis_BB2 : Outport
  wires:
  <IP_LB_BMS_DYN_Lim_Current_OUT_A_DataBus>/1 -> Bus Selector1/1
  Bus Selector1/1 -> Multiport Switch/3  "<sData>"
  [Select_Battery2] -> Multiport Switch/1
  <IP_sBatt2_DisChargeCurrentMax_A_Databus>/1 -> Bus Selector/1
  Constant/1 -> Multiport Switch/5, Multiport Switch/4
  Multiport Switch/1 -> IP_sBMS_DisChargeCurrentPrognosis_BB2/1  "IP_sBMS_DisChargeCurrentPrognosis_BB2"
  Bus Selector/1 -> Multiport Switch/2  "<sData>"

== system ChiefMaster_TTC580/ChiefMaster/Input Translation/Battery Signals/Subsystem4/Subsystem2 ==
  <IP_sBatt3_DisChargeCurrentMax_A_Databus> : Inport
  <IP_LB_BMS_DYN_Lim_Current_OUT_A_DataBus> : Inport  Port=2
  Bus Selector : BusSelector  OutputSignals=sData
  Bus Selector1 : BusSelector  OutputSignals=sData
  Constant : Constant  Value=0  OutDataTypeStr=single
  Multiport Switch : MultiPortSwitch  DataPortForDefault=Additional data port  DiagnosticForDefault=Warning  SaturateOnIntegerOverflow=off  InputSameDT=off
  IP_sBMS_DisChargeCurrentPrognosis_BB2 : Outport
  wires:
  Bus Selector/1 -> Multiport Switch/2  "<sData>"
  Multiport Switch/1 -> IP_sBMS_DisChargeCurrentPrognosis_BB2/1  "IP_sBMS_DisChargeCurrentPrognosis_BB2"
  Constant/1 -> Multiport Switch/4, Multiport Switch/5
  <IP_sBatt3_DisChargeCurrentMax_A_Databus>/1 -> Bus Selector/1
  [Select_Battery3] -> Multiport Switch/1
  Bus Selector1/1 -> Multiport Switch/3  "<sData>"
  <IP_LB_BMS_DYN_Lim_Current_OUT_A_DataBus>/1 -> Bus Selector1/1

== system ChiefMaster_TTC580/ChiefMaster/Input Translation/Battery Signals/Subsystem5/Subsystem ==
  <IP_sBatt1_ChargeCurrentMax_A_Databus> : Inport
  <IP_LB_BMS_REQ_Charger_Current_A_DataBus> : Inport  Port=2
  <IP_LB_BMS_DYN_Lim_Current_IN_A_DataBus> : Inport  Port=3
  Bus Selector : BusSelector  OutputSignals=sData
  Bus Selector1 : BusSelector  OutputSignals=sData
  Bus Selector2 : BusSelector  OutputSignals=sData
  Constant : Constant  Value=0  OutDataTypeStr=single
  Min : MinMax  Inputs=2
  Multiport Switch : MultiPortSwitch  DataPortForDefault=Additional data port  DiagnosticForDefault=Warning  SaturateOnIntegerOverflow=off  InputSameDT=off
  IP_sBMS_ChargeCurrentPrognosis_BB1 : Outport
  wires:
  <IP_LB_BMS_REQ_Charger_Current_A_DataBus>/1 -> Bus Selector1/1
  Bus Selector1/1 -> Min/1  "<sData>"
  [Select_Battery1] -> Multiport Switch/1
  <IP_sBatt1_ChargeCurrentMax_A_Databus>/1 -> Bus Selector/1
  <IP_LB_BMS_DYN_Lim_Current_IN_A_DataBus>/1 -> Bus Selector2/1
  Constant/1 -> Multiport Switch/5, Multiport Switch/4
  Multiport Switch/1 -> IP_sBMS_ChargeCurrentPrognosis_BB1/1  "IP_sBMS_ChargeCurrentPrognosis_BB1"
  Bus Selector/1 -> Multiport Switch/2  "<sData>"
  Bus Selector2/1 -> Min/2  "<sData>"
  Min/1 -> Multiport Switch/3

== system ChiefMaster_TTC580/ChiefMaster/Input Translation/Battery Signals/Subsystem5/Subsystem1 ==
  <IP_sBatt2_ChargeCurrentMax_A_Databus> : Inport
  <IP_LB_BMS_REQ_Charger_Current_A_DataBus> : Inport  Port=2
  <IP_LB_BMS_DYN_Lim_Current_IN_A_DataBus> : Inport  Port=3
  Bus Selector : BusSelector  OutputSignals=sData
  Bus Selector1 : BusSelector  OutputSignals=sData
  Bus Selector2 : BusSelector  OutputSignals=sData
  Constant : Constant  Value=0  OutDataTypeStr=single
  Min : MinMax  Inputs=2
  Multiport Switch : MultiPortSwitch  DataPortForDefault=Additional data port  DiagnosticForDefault=Warning  SaturateOnIntegerOverflow=off  InputSameDT=off
  IP_sBMS_ChargeCurrentPrognosis_BB2 : Outport
  wires:
  Bus Selector2/1 -> Min/2  "<sData>"
  Bus Selector/1 -> Multiport Switch/2  "<sData>"
  Multiport Switch/1 -> IP_sBMS_ChargeCurrentPrognosis_BB2/1  "IP_sBMS_ChargeCurrentPrognosis_BB2"
  Constant/1 -> Multiport Switch/4, Multiport Switch/5
  <IP_LB_BMS_DYN_Lim_Current_IN_A_DataBus>/1 -> Bus Selector2/1
  <IP_sBatt2_ChargeCurrentMax_A_Databus>/1 -> Bus Selector/1
  [Select_Battery2] -> Multiport Switch/1
  Bus Selector1/1 -> Min/1  "<sData>"
  <IP_LB_BMS_REQ_Charger_Current_A_DataBus>/1 -> Bus Selector1/1
  Min/1 -> Multiport Switch/3

== system ChiefMaster_TTC580/ChiefMaster/Input Translation/Battery Signals/Subsystem5/Subsystem2 ==
  <IP_sBatt3_ChargeCurrentMax_A_Databus> : Inport
  <IP_LB_BMS_REQ_Charger_Current_A_DataBus> : Inport  Port=2
  <IP_LB_BMS_DYN_Lim_Current_IN_A_DataBus> : Inport  Port=3
  Bus Selector : BusSelector  OutputSignals=sData
  Bus Selector1 : BusSelector  OutputSignals=sData
  Bus Selector2 : BusSelector  OutputSignals=sData
  Constant : Constant  Value=0  OutDataTypeStr=single
  Min : MinMax  Inputs=2
  Multiport Switch : MultiPortSwitch  DataPortForDefault=Additional data port  DiagnosticForDefault=Warning  SaturateOnIntegerOverflow=off  InputSameDT=off
  IP_sBMS_ChargeCurrentPrognosis_BB2 : Outport
  wires:
  <IP_LB_BMS_DYN_Lim_Current_IN_A_DataBus>/1 -> Bus Selector2/1
  <IP_LB_BMS_REQ_Charger_Current_A_DataBus>/1 -> Bus Selector1/1
  <IP_sBatt3_ChargeCurrentMax_A_Databus>/1 -> Bus Selector/1
  Bus Selector1/1 -> Min/1  "<sData>"
  [Select_Battery3] -> Multiport Switch/1
  Constant/1 -> Multiport Switch/5, Multiport Switch/4
  Multiport Switch/1 -> IP_sBMS_ChargeCurrentPrognosis_BB2/1  "IP_sBMS_ChargeCurrentPrognosis_BB3"
  Bus Selector/1 -> Multiport Switch/2  "<sData>"
  Bus Selector2/1 -> Min/2  "<sData>"
  Min/1 -> Multiport Switch/3

== system ChiefMaster_TTC580/ChiefMaster/Input Translation/Battery Signals/Subsystem6/Subsystem3 ==
  <IP_sBatt1_Current_A_DataBus> : Inport
  <IP_LB_BMS_Pack_Current_Master_mA_DataBus> : Inport  Port=2
  Bus Selector1 : BusSelector  OutputSignals=sData
  Bus Selector7 : BusSelector  OutputSignals=sData
  Constant : Constant  Value=0  OutDataTypeStr=single
  Multiport Switch : MultiPortSwitch  DataPortForDefault=Additional data port  DiagnosticForDefault=Warning  SaturateOnIntegerOverflow=off  InputSameDT=off
  mAtoA : Gain  Gain=1/1000
  IP_sBMS_Current_BB1 : Outport
  wires:
  Bus Selector1/1 -> mAtoA/1  "<sData>"
  Bus Selector7/1 -> Multiport Switch/2  "<sData>"
  <IP_sBatt1_Current_A_DataBus>/1 -> Bus Selector7/1
  <IP_LB_BMS_Pack_Current_Master_mA_DataBus>/1 -> Bus Selector1/1
  Constant/1 -> Multiport Switch/4, Multiport Switch/5
  mAtoA/1 -> Multiport Switch/3
  [Select_Battery1] -> Multiport Switch/1
  Multiport Switch/1 -> IP_sBMS_Current_BB1/1  "IP_sBMS_Current_BB1"

== system ChiefMaster_TTC580/ChiefMaster/Input Translation/Battery Signals/Subsystem6/Subsystem4 ==
  <IP_sBatt2_Current_A_DataBus> : Inport
  <IP_LB_BMS_Pack_Current_Master_mA_DataBus> : Inport  Port=2
  Bus Selector1 : BusSelector  OutputSignals=sData
  Bus Selector7 : BusSelector  OutputSignals=sData
  Constant : Constant  Value=0  OutDataTypeStr=single
  Multiport Switch : MultiPortSwitch  DataPortForDefault=Additional data port  DiagnosticForDefault=Warning  SaturateOnIntegerOverflow=off  InputSameDT=off
  mAtoA : Gain  Gain=1/1000
  IP_sBMS_Current_BB2 : Outport
  wires:
  Multiport Switch/1 -> IP_sBMS_Current_BB2/1  "IP_sBMS_Current_BB2"
  [Select_Battery2] -> Multiport Switch/1
  mAtoA/1 -> Multiport Switch/3
  Constant/1 -> Multiport Switch/5, Multiport Switch/4
  <IP_LB_BMS_Pack_Current_Master_mA_DataBus>/1 -> Bus Selector1/1
  <IP_sBatt2_Current_A_DataBus>/1 -> Bus Selector7/1
  Bus Selector7/1 -> Multiport Switch/2  "<sData>"
  Bus Selector1/1 -> mAtoA/1  "<sData>"

== system ChiefMaster_TTC580/ChiefMaster/Input Translation/Battery Signals/Subsystem6/Subsystem5 ==
  <IP_sBatt3_Current_A_DataBus> : Inport
  <IP_LB_BMS_Pack_Current_Master_mA_DataBus> : Inport  Port=2
  Bus Selector1 : BusSelector  OutputSignals=sData
  Bus Selector7 : BusSelector  OutputSignals=sData
  Constant : Constant  Value=0  OutDataTypeStr=single
  Multiport Switch : MultiPortSwitch  DataPortForDefault=Additional data port  DiagnosticForDefault=Warning  SaturateOnIntegerOverflow=off  InputSameDT=off
  mAtoA : Gain  Gain=1/1000
  IP_sBMS_Current_BB3 : Outport
  wires:
  Bus Selector1/1 -> mAtoA/1  "<sData>"
  Bus Selector7/1 -> Multiport Switch/2  "<sData>"
  Constant/1 -> Multiport Switch/4, Multiport Switch/5
  mAtoA/1 -> Multiport Switch/3
  [Select_Battery3] -> Multiport Switch/1
  Multiport Switch/1 -> IP_sBMS_Current_BB3/1  "IP_sBMS_Current_BB3"
  <IP_sBatt3_Current_A_DataBus>/1 -> Bus Selector7/1
  <IP_LB_BMS_Pack_Current_Master_mA_DataBus>/1 -> Bus Selector1/1

== system ChiefMaster_TTC580/ChiefMaster/Input Translation/Battery Signals/Subsystem7/Subsystem1 ==
  <IP_boBatt2_Insulation_ready_and_OK> : Inport
  IP_LiBa_Insulation_OK_BB2 : Inport  Port=2
  IMD_Req_Databus : Inport  Port=3
  Bus Selector : BusSelector  OutputSignals=FL_IMD_Control_Databus.FL_boREQ_IMD_ON_BB1
  Constant : Constant  Value=0  OutDataTypeStr=boolean
  Constant1 : Constant  Value=IT_u8IMD_DelayTime_s  OutDataTypeStr=uint8
  Delay : Delay  DelayLength=3
  IMD_OK : Stateflow chart  TreatAsAtomicUnit=on
  Multiport Switch : MultiPortSwitch  DataPortForDefault=Additional data port  DiagnosticForDefault=Warning  SaturateOnIntegerOverflow=off  InputSameDT=off
  IP_boBMS_InsulationReadyOK_B2 : Outport  OutDataTypeStr=boolean
  wires:
  Multiport Switch/1 -> IP_boBMS_InsulationReadyOK_B2/1  "IP_boBMS_InsulationReadyOK_B2"
  <IP_boBatt2_Insulation_ready_and_OK>/1 -> Multiport Switch/2
  [Select_Battery2] -> Multiport Switch/1
  IP_LiBa_Insulation_OK_BB2/1 -> IMD_OK/1(IP_boBMS_InsulationReadyOK)
  Constant/1 -> Multiport Switch/4, Multiport Switch/5
  IMD_OK/1(IMD_OK) -> Multiport Switch/3
  IMD_Req_Databus/1 -> Bus Selector/1
  Bus Selector/1 -> Delay/1  "<FL_boREQ_IMD_ON_BB1>"
  Delay/1 -> IMD_OK/2(Req_IMD)
  Constant1/1 -> IMD_OK/3(IT_u8IMD_DelayTime_s)

== system ChiefMaster_TTC580/ChiefMaster/Input Translation/Battery Signals/Subsystem7/Subsystem2 ==
  <IP_boBatt3_Insulation_ready_and_OK> : Inport
  IP_LiBa_Insulation_OK_BB3 : Inport  Port=2
  IMD_Req_Databus : Inport  Port=3
  Bus Selector : BusSelector  OutputSignals=FL_IMD_Control_Databus.FL_boREQ_IMD_ON_BB1
  Constant : Constant  Value=0  OutDataTypeStr=boolean
  Constant1 : Constant  Value=IT_u8IMD_DelayTime_s  OutDataTypeStr=uint8
  Delay : Delay  DelayLength=3
  IMD_OK : Stateflow chart  TreatAsAtomicUnit=on
  Multiport Switch : MultiPortSwitch  DataPortForDefault=Additional data port  DiagnosticForDefault=Warning  SaturateOnIntegerOverflow=off  InputSameDT=off
  IP_boBMS_InsulationReadyOK_B3 : Outport  OutDataTypeStr=boolean
  wires:
  Constant/1 -> Multiport Switch/5, Multiport Switch/4
  IP_LiBa_Insulation_OK_BB3/1 -> IMD_OK/1(IP_boBMS_InsulationReadyOK)
  [Select_Battery3] -> Multiport Switch/1
  <IP_boBatt3_Insulation_ready_and_OK>/1 -> Multiport Switch/2
  Multiport Switch/1 -> IP_boBMS_InsulationReadyOK_B3/1  "IP_boBMS_InsulationReadyOK_B3"
  IMD_OK/1(IMD_OK) -> Multiport Switch/3
  IMD_Req_Databus/1 -> Bus Selector/1
  Bus Selector/1 -> Delay/1  "<FL_boREQ_IMD_ON_BB1>"
  Delay/1 -> IMD_OK/2(Req_IMD)
  Constant1/1 -> IMD_OK/3(IT_u8IMD_DelayTime_s)

== system ChiefMaster_TTC580/ChiefMaster/Input Translation/Battery Signals/Subsystem7/Subsystem3 ==
  <IP_boBatt1_Insulation_ready_and_OK> : Inport
  IP_LiBa_Insulation_OK_BB1 : Inport  Port=2
  IMD_Req_Databus : Inport  Port=3
  Bus Selector : BusSelector  OutputSignals=FL_IMD_Control_Databus.FL_boREQ_IMD_ON_BB1
  Constant : Constant  Value=0  OutDataTypeStr=boolean
  Constant1 : Constant  Value=IT_u8IMD_DelayTime_s  OutDataTypeStr=uint8
  Delay : Delay  DelayLength=3
  IMD_OK : Stateflow chart  TreatAsAtomicUnit=on
  Multiport Switch : MultiPortSwitch  DataPortForDefault=Additional data port  DiagnosticForDefault=Warning  SaturateOnIntegerOverflow=off  InputSameDT=off
  IP_boBMS_InsulationReadyOK_B1 : Outport  OutDataTypeStr=boolean
  wires:
  Constant/1 -> Multiport Switch/5, Multiport Switch/4
  [Select_Battery1] -> Multiport Switch/1
  <IP_boBatt1_Insulation_ready_and_OK>/1 -> Multiport Switch/2
  Multiport Switch/1 -> IP_boBMS_InsulationReadyOK_B1/1  "IP_boBMS_InsulationReadyOK_B1"
  IP_LiBa_Insulation_OK_BB1/1 -> IMD_OK/1(IP_boBMS_InsulationReadyOK)
  IMD_OK/1(IMD_OK) -> Multiport Switch/3
  Bus Selector/1 -> Delay/1  "<FL_boREQ_IMD_ON_BB1>"
  Delay/1 -> IMD_OK/2(Req_IMD)
  IMD_Req_Databus/1 -> Bus Selector/1
  Constant1/1 -> IMD_OK/3(IT_u8IMD_DelayTime_s)

== system ChiefMaster_TTC580/ChiefMaster/Input Translation/Battery Signals/Subsystem8/Subsystem ==
  <IP_sBatt1_Availability> : Inport
  <IP_sLiBa_Batt1_Availability> : Inport  Port=2
  Constant : Constant  Value=0  OutDataTypeStr=boolean
  Multiport Switch : MultiPortSwitch  DataPortForDefault=Additional data port  DiagnosticForDefault=Warning  SaturateOnIntegerOverflow=off  InputSameDT=off
  IP_boBMS_Batt1_Availability : Outport
  wires:
  Multiport Switch/1 -> IP_boBMS_Batt1_Availability/1  "IP_boBMS_Batt1_Availability"
  [Select_Battery1] -> Multiport Switch/1
  Constant/1 -> Multiport Switch/4, Multiport Switch/5
  <IP_sBatt1_Availability>/1 -> Multiport Switch/2
  <IP_sLiBa_Batt1_Availability>/1 -> Multiport Switch/3

== system ChiefMaster_TTC580/ChiefMaster/Input Translation/Battery Signals/Subsystem8/Subsystem1 ==
  <IP_sBatt2_Availability> : Inport
  <IP_sLiBa_Batt2_Availability> : Inport  Port=2
  Constant : Constant  Value=0  OutDataTypeStr=boolean
  Multiport Switch : MultiPortSwitch  DataPortForDefault=Additional data port  DiagnosticForDefault=Warning  SaturateOnIntegerOverflow=off  InputSameDT=off
  IP_boBMS_Batt2_Availability : Outport
  wires:
  <IP_sLiBa_Batt2_Availability>/1 -> Multiport Switch/3
  <IP_sBatt2_Availability>/1 -> Multiport Switch/2
  Constant/1 -> Multiport Switch/5, Multiport Switch/4
  [Select_Battery2] -> Multiport Switch/1
  Multiport Switch/1 -> IP_boBMS_Batt2_Availability/1  "IP_boBMS_Batt2_Availability"

== system ChiefMaster_TTC580/ChiefMaster/Input Translation/Battery Signals/Subsystem8/Subsystem2 ==
  <IP_sBatt3_Availability> : Inport
  <IP_sLiBa_Batt3_Availability> : Inport  Port=2
  Constant : Constant  Value=0  OutDataTypeStr=boolean
  Multiport Switch : MultiPortSwitch  DataPortForDefault=Additional data port  DiagnosticForDefault=Warning  SaturateOnIntegerOverflow=off  InputSameDT=off
  IP_boBMS_Batt3_Availability : Outport
  wires:
  Multiport Switch/1 -> IP_boBMS_Batt3_Availability/1  "IP_boBMS_Batt3_Availability"
  [Select_Battery3] -> Multiport Switch/1
  Constant/1 -> Multiport Switch/4, Multiport Switch/5
  <IP_sBatt3_Availability>/1 -> Multiport Switch/2
  <IP_sLiBa_Batt3_Availability>/1 -> Multiport Switch/3

== system ChiefMaster_TTC580/ChiefMaster/Input Translation/Battery Signals/Subsystem9/Subsystem1 ==
  <IP_LB_BMS_IO_state_Input_DataBus> : Inport
  <IP_boBatt1_HV_relay_PLUS_Sense> : Inport  Port=2
  Bus Selector : BusSelector  OutputSignals=sData
  Compare To Constant : simulink/Logic and Bit Operations/Compare To Constant  relop===  const=128  OutDataTypeStr=boolean
  Compare To Constant1 : simulink/Logic and Bit Operations/Compare To Constant  relop===  const=160  OutDataTypeStr=boolean
  Compare To Constant2 : simulink/Logic and Bit Operations/Compare To Constant  relop===  const=224  OutDataTypeStr=boolean
  Constant : Constant  Value=0  OutDataTypeStr=boolean
  Multiport Switch : MultiPortSwitch  DataPortForDefault=Additional data port  DiagnosticForDefault=Warning  SaturateOnIntegerOverflow=off  InputSameDT=off
  OR : Logic  Operator=OR  Inputs=3  AllPortsSameDT=off  OutDataTypeStr=boolean
  IP_boBMS_HV_Plus_Sense_BB1 : Outport
  wires:
  <IP_LB_BMS_IO_state_Input_DataBus>/1 -> Bus Selector/1
  <IP_boBatt1_HV_relay_PLUS_Sense>/1 -> Multiport Switch/2
  Constant/1 -> Multiport Switch/5, Multiport Switch/4
  [Select_Battery1] -> Multiport Switch/1
  Multiport Switch/1 -> IP_boBMS_HV_Plus_Sense_BB1/1  "IP_boBMS_HV_Plus_Sense_BB1"
  Compare To Constant1/1 -> OR/2
  Bus Selector/1 -> Compare To Constant/1, Compare To Constant2/1, Compare To Constant1/1  "<sData>"
  Compare To Constant/1 -> OR/1
  OR/1 -> Multiport Switch/3
  Compare To Constant2/1 -> OR/3
